simulink model "rlVarth"  (R2020b)
settings: Solver=ode23t  StartTime=0.0  StopTime=Tf  RelTol=1e-2
model workspace: external: MAT-File C:\PhD\Variable Threshold\demo_rl.mat (data not in the file)
values from neighbouring files (symbols this model uses):
  actorAtk = rlDeterministicActorRepresentation(actorNetwork,obsInfo{1,1},actInfo{1,1},'Observation',{'State'},'Action',{'Action'},actorOptions)    [demo_rl.m]    (also in main_rl.m = rlDeterministicActorRepresentation(actorNetwork,obsInfo{1,1}; main_rl_func_modified.m = rlDeterministicActorRepresentation(actorNetwork,obsInfo{1,1}; new_main_rl.m = rlDeterministicActorRepresentation(actorNetwork,obsInfo{1,1})
  actorCon = rlDeterministicActorRepresentation(actorNetwork,obsInfo{1,2},actInfo{1,2},'Observation',{'State'},'Action',{'Action'},actorOptions)    [demo_rl.m]    (also in main_rl.m = rlDeterministicActorRepresentation(actorNetwork,obsInfo{1,2}; main_rl_func_modified.m = rlDeterministicActorRepresentation(actorNetwork,obsInfo{1,2}; new_main_rl.m = rlDeterministicActorRepresentation(actorNetwork,obsInfo{1,2})
  actorDtc = rlDeterministicActorRepresentation(actorNetwork,obsInfo{1,3},actInfo{1,3},'Observation',{'State'},'Action',{'Action'},actorOptions)    [demo_rl.m]    (also in main_rl.m = rlDeterministicActorRepresentation(actorNetwork,obsInfo{1,3}; main_rl_func_modified.m = rlDeterministicActorRepresentation(actorNetwork,obsInfo{1,3}; new_main_rl.m = rlDeterministicActorRepresentation(actorNetwork,obsInfo{1,3})
  agentOpts = rlDDPGAgentOptions(     'SampleTime',Ts,     'TargetSmoothFactor',1e-3,     'DiscountFactor',1.0,      'MiniBatchSize',64,      'ExperienceBufferLength',1e6)    [demo_rl.m]    (also in main_rl.m = rlDDPGAgentOptions(     'SampleTime',Ts,     'TargetSmoothFa; main_rl_func_modified.m = rlDDPGAgentOptions(     'SampleTime',Ts,     'TargetSmoothFa; new_main_rl.m = rlDDPGAgentOptions(     'SampleTime',Ts,     'TargetSmoothFa)
  criticAtk = rlQValueRepresentation(criticNetwork,obsInfo{1,1},actInfo{1,1},'Observation',{'State'},'Action',{'Action'},criticOpts)    [demo_rl.m]    (also in main_rl.m = rlQValueRepresentation(criticNetwork,obsInfo{1,1},actInfo{1,; main_rl_func_modified.m = rlQValueRepresentation(criticNetwork,obsInfo{1,1},actInfo{1,; new_main_rl.m = rlQValueRepresentation(criticNetwork,obsInfo{1,1},actInfo{1,)
  criticCon = rlQValueRepresentation(criticNetwork,obsInfo{1,2},actInfo{1,2},'Observation',{'State'},'Action',{'Action'},criticOpts)    [demo_rl.m]    (also in main_rl.m = rlQValueRepresentation(criticNetwork,obsInfo{1,2},actInfo{1,; main_rl_func_modified.m = rlQValueRepresentation(criticNetwork,obsInfo{1,2},actInfo{1,; new_main_rl.m = rlQValueRepresentation(criticNetwork,obsInfo{1,2},actInfo{1,)
  criticDtc = rlQValueRepresentation(criticNetwork,obsInfo{1,3},actInfo{1,3},'Observation',{'State'},'Action',{'Action'},criticOpts)    [demo_rl.m]    (also in main_rl.m = rlQValueRepresentation(criticNetwork,obsInfo{1,3},actInfo{1,; main_rl_func_modified.m = rlQValueRepresentation(criticNetwork,obsInfo{1,3},actInfo{1,; new_main_rl.m = rlQValueRepresentation(criticNetwork,obsInfo{1,3},actInfo{1,)
  Tf = 200    [RLenv.m]    (also in RlEnvModel.m; demo_rl.m; main_rl.m = simlen*Ts; main_rl_func_modified.m = simlen*Ts)
  Ts = 0.1    [RLenv.m]    (also in RlEnvModel.m; demo_rl.m; main_rl.m = s.Ts; main_rl_func_modified.m = s.Ts)
undefined symbols (not defined in the file or in its folder): esp_env, rlDDPGAgent
libraries: rllib x3, simulink x2
settings Model: Creator=The MathWorks, Inc.  LastModifiedBy=IIT_KGP_CSE_FM_LAB

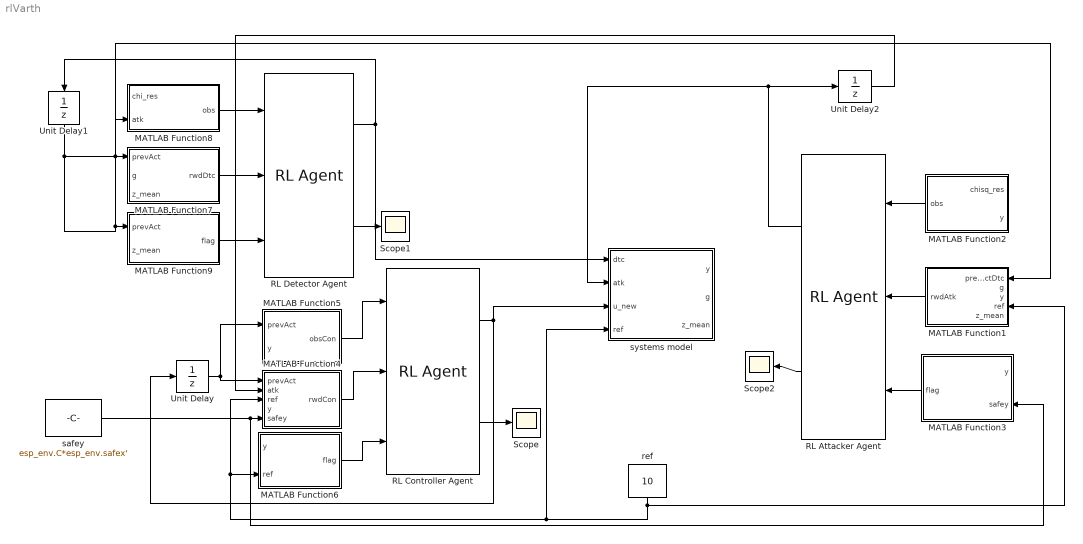
== system rlVarth ==
  MATLAB Function1 : MATLAB Function  TreatAsAtomicUnit=on
  MATLAB Function2 : MATLAB Function  TreatAsAtomicUnit=on
  MATLAB Function3 : MATLAB Function  TreatAsAtomicUnit=on
  MATLAB Function4 : MATLAB Function  TreatAsAtomicUnit=on
  MATLAB Function5 : MATLAB Function  TreatAsAtomicUnit=on
  MATLAB Function6 : MATLAB Function  TreatAsAtomicUnit=on
  MATLAB Function7 : MATLAB Function  TreatAsAtomicUnit=on
  MATLAB Function8 : MATLAB Function  TreatAsAtomicUnit=on
  MATLAB Function9 : MATLAB Function  TreatAsAtomicUnit=on
  RL Attacker Agent : rllib/RL Agent  Agent=rlDDPGAgent(actorAtk,criticAtk,agentOpts)  ProvideReward=on  ProvideIsDone=on  ProvideCumRwd=on  TreatAsDirectFeedthrough=on  CollectLoggedSignals=on  CollectModelStates=on
  RL Controller Agent : rllib/RL Agent  Agent=rlDDPGAgent(actorCon,criticCon,agentOpts)  ProvideReward=on  ProvideIsDone=on  ProvideCumRwd=on  TreatAsDirectFeedthrough=on  CollectLoggedSignals=on  CollectModelStates=on
  RL Detector Agent : rllib/RL Agent  Agent=rlDDPGAgent(actorDtc,criticDtc,agentOpts)  ProvideReward=on  ProvideIsDone=on  ProvideCumRwd=on  TreatAsDirectFeedthrough=on  CollectLoggedSignals=on  CollectModelStates=on
  Scope : Scope
  Scope1 : Scope
  Scope2 : Scope
  Unit Delay : UnitDelay  SampleTime=-1  HasFrameUpgradeWarning=on
  Unit Delay1 : UnitDelay  SampleTime=-1  HasFrameUpgradeWarning=on
  Unit Delay2 : UnitDelay  SampleTime=-1  HasFrameUpgradeWarning=on
  ref : Constant  Value=10
  safey : Constant  Value=esp_env.C*esp_env.safex'
  systems model : Subsystem
  wires:
  RL Attacker Agent/1 -> systems model/2(atk), Unit Delay2/1
  MATLAB Function2/1(obs) -> RL Attacker Agent/1
  ref/1 -> systems model/4(ref), MATLAB Function4/3(ref), MATLAB Function6/2(ref), MATLAB Function1/4(ref)
  MATLAB Function1/1(rwdAtk) -> RL Attacker Agent/2
  MATLAB Function3/1(flag) -> RL Attacker Agent/3
  MATLAB Function5/1(obsCon) -> RL Controller Agent/1
  MATLAB Function4/1(rwdCon) -> RL Controller Agent/2
  MATLAB Function6/1(flag) -> RL Controller Agent/3
  RL Controller Agent/1 -> Unit Delay/1, systems model/3(u_new)
  MATLAB Function8/1(obs) -> RL Detector Agent/1
  MATLAB Function9/1(flag) -> RL Detector Agent/3
  MATLAB Function7/1(rwdDtc) -> RL Detector Agent/2
  RL Detector Agent/1 -> systems model/1(dtc), Unit Delay1/1
  RL Controller Agent/2 -> Scope/1
  RL Detector Agent/2 -> Scope1/1
  RL Attacker Agent/2 -> Scope2/1
  Unit Delay/1 -> MATLAB Function4/1(prevAct), MATLAB Function5/1(prevAct)
  Unit Delay1/1 -> MATLAB Function8/2(atk), MATLAB Function7/1(prevAct), MATLAB Function1/1(prevActDtc), MATLAB Function9/1(prevAct)
  ? -> MATLAB Function3/1(y), MATLAB Function2/2(y), MATLAB Function1/3(y), MATLAB Function6/1(y), MATLAB Function5/2(y), MATLAB Function4/4(y), MATLAB Function1/5(z_mean), MATLAB Function8/1(chi_res), MATLAB Function7/2(g), MATLAB Function1/2(g), MATLAB Function2/1(chisq_res), MATLAB Function9/2(z_mean), MATLAB Function7/3(z_mean)
  Unit Delay2/1 -> MATLAB Function4/2(atk)
  safey/1 -> MATLAB Function3/2(safey), MATLAB Function4/5(safey)

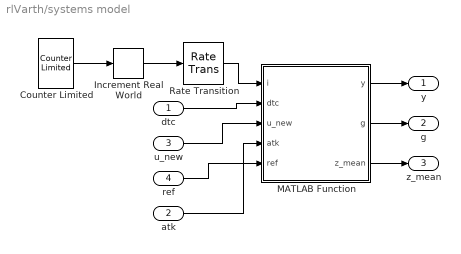
== system rlVarth/systems model ==
  dtc : Inport
  atk : Inport  Port=2
  u_new : Inport  Port=3
  ref : Inport  Port=4
  Counter Limited : simulink/Sources/Counter Limited  uplimit=Tf/Ts  tsamp=Ts
  Increment Real World : simulink/Additional Math & Discrete/Additional Math: Increment - Decrement/Increment Real World
      settings: SourceProductBaseCode=SL
  MATLAB Function : MATLAB Function  TreatAsAtomicUnit=on
  Rate Transition : RateTransition
  y : Outport
  g : Outport  Port=2
  z_mean : Outport  Port=3
  wires:
  MATLAB Function/3(z_mean) -> z_mean/1
  MATLAB Function/2(g) -> g/1
  Increment Real World/1 -> Rate Transition/1
  MATLAB Function/1(y) -> y/1
  atk/1 -> MATLAB Function/4(atk)
  Rate Transition/1 -> MATLAB Function/1(i)
  Counter Limited/1 -> Increment Real World/1
  dtc/1 -> MATLAB Function/2(dtc)
  u_new/1 -> MATLAB Function/3(u_new)
  ref/1 -> MATLAB Function/5(ref)

== matlab function rlVarth/MATLAB Function9 ==
  data: prevAct input; flag output; z_mean input
function flag  = stopDtc(prevAct,z_mean)
   th= prevAct(1);
   tau = prevAct(2,1);
   dof = size(y,1)*(tau);
   FAR = 1-chi2cdf(th,dof);
   TPR = 1- ncx2cdf(th,dof,z_mean)
   if FAR < 0.004 & TPR > 0.96
       flag=1;
   end

== matlab function rlVarth/MATLAB Function1 ==
  data: rwdAtk output; prevActDtc input; g input; y input; ref input; z_mean input
function rwdAtk  = rwrdAtk(prevActDtc,g,y,ref,z_mean)
   th= prevActDtc(1);
   tau = prevActDtc(2,1);
   dof = size(y,1)*(tau);
   FAR = 1-chi2cdf(th,dof);
   TPR = 1- ncx2cdf(th,dof,z_mean)
   rwdAtk = FAR/TPR + 50*(g<th)+ 100*(y-ref)^2;

== matlab function rlVarth/systems model/MATLAB Function ==
  data: i input; y output; g output; z_mean output; dtc input; u_new input; atk input; ref input; s parameter
function [y,g,z_mean] = env(i,dtc,u_new,atk,ref, s)
% function [y,g,z_mean]= envSys(atk,dtc,new_u,ref, s)
%% SYS_ENV Summary of this function goes here

%%%%%%%%%%%%%%%%%%%%%%%%%%%=====FDI Attack=========%%%%%%%%%%%%%%%%%%%%%
%========================== obtained from code ======================%
% x1_0=-15.0;
% x2_0=16.6096079397;
% fdi_u=[ 35.99313719  71.98627437  58.33575204  41.29588025   0.   0.         -31.21892088  -5.09118639   0.           0.  -0.41831677   0.           0.           0.           0.   0. ];
% fdi_y=[15.01515367 13.48175215 11.26355514 10.30553807  8.22658704  4.85366237  3.61911687  2.21566942  1.21608204  0.53164255  0.1748743   0.  0.          0.          0.          0. ];
%======================================================================%

% ay=  [fdi_y,zeros(1,time-size(fdi_y,2))];
% au = [fdi_u,zeros(1,time-size(fdi_u,2))];

%%%%%%%%%%%%%%%%%%%%%%%%%%=====System Simulation======%%%%%%%%%%%%%%%%%%

%====================Chi Squared Test =================
% tau = 1; % Detection window % new: let's check for every iteration now
%======================================================
% stateProg(esp_env,i,dtc(2),dtc(1),new_u,atk(1),atk(2))
au= atk(1);

ay= atk(2);
th= dtc(1);
tau= dtc(2);
% coder.extrinsic('evalin','assignin');
% evalin
%  for i = 1:esp_env.Ts:esp_env.Tf
    
    
            s.t(i+1)=i*s.Ts;
            s.a_u(:,i+1)=au;
            s.a_y(:,i+1)=ay;
            s.x_act(:,i+1) = s.A*s.x_act(i)+s.B*s.uatk(i)+s.proc_noise(i);
%             s.xatk(i)= s.A*s.x_act(i)+s.B*s.u_act(i);
            s.xhat(:,i+1) = s.A*s.xhat(i) + s.B*s.u_act(i) + s.L*s.z(i);
            s.est_err(:,i+1)= s.x_act(:,i+1)-s.xhat(:,i+1);
            s.u_act(:,i+1)= s.K*s.xhat(:,i+1);
            s.uatk(:,i+1)= s.u_act(:,i+1)+s.a_u(:,i+1);
            s.y_act(:,i+1)= s.C*s.x_act(i+1)+s.meas_noise(i);
            s.yatk(:,i+1)= s.y_act(:,i+1)+s.a_y(:,i+1);
            s.z(:,i+1)= s.yatk(:,i+1)-C*s.xhat(:,i+1);
            s.z_mean(:,i+1)= mean(s.z);
            s.P = cov(s.z');
            s.chi_tst(i+1)= z(:,i+1)'*inv(P)*z(:,i+1);
            s.threshold(i+1)= th;
            s.tau(i+1)= dtc_windw;
            s.g(i+1) = 0;               
%             if i-tau+1 > 0                  % Calculate detector window starting index
%                 srt = i-tau+1;              % tau is the detector window length
%             else
%                 srt = 1;
%             end
            for k = max(1,i-s.tau(i+1)+1):i+1
                s.g(i+1) = s.g(i+1) + s.chi_tst(k);  % Calculate gk (chi2 test)
            end
            if s.g(i+1) > s.threshold(i+1)
                s.u_act(:,i+1) = u_new;
                s.uatk(:,i+1)= s.u_act(:,i+1)+s.a_u(:,i+1);
                isatk=1;
            else
                isatk=0;
            end

    g= s.g(i+1);
    y=s.yatk(:,i+1);
    z_mean = s.z_mean(i+1);

end

== matlab function rlVarth/MATLAB Function2 ==
  data: obs output; chisq_res input; y input
function obs = obsAtk(chisq_res,y)
    obs= [chi_sq,y];

== matlab function rlVarth/MATLAB Function3 ==
  data: y input; flag output; safey input
function flag  = stop(y,safey)
    flag = y >safey;

== matlab function rlVarth/MATLAB Function4 ==
  data: rwdCon output; prevAct input; atk input; ref input; y input; safey input
function rwdCon  = rwrdCon(prevAct,atk,ref,y,safey)
    au=atk(1);
    ay=atk(2);
    rwdCon = -(prevAct+au)^2-20*(y-ref)^2-200*(abs(y) > safey);

== matlab function rlVarth/MATLAB Function5 ==
  data: obsCon output; prevAct input; y input
function obsCon = obsCon(prevAct,y)
   
    obsCon=[prevAct,y];

== matlab function rlVarth/MATLAB Function6 ==
  data: y input; ref input; flag output
function flag  = stop(y,ref)
    
    flag= abs(y-ref) == 0;

== matlab function rlVarth/MATLAB Function7 ==
  data: rwdDtc output; prevAct input; g input; z_mean input
function rwdDtc  = rwrdDtc(prevAct,g,z_mean)
   th= prevAct(1);
   tau = prevAct(2,1);
   dof = size(y,1)*(tau);
   FAR = 1-chi2cdf(th,dof);
   TPR = 1- ncx2cdf(th,dof,z_mean)
   rwdDtc = TPR/FAR + 50*(g<=th);

== matlab function rlVarth/MATLAB Function8 ==
  data: obs output; chi_res input; atk input
function obs = obsDtc(chi_res,atk)
   
    obs=[chi_res,atk];
